simulink model "Closed_loop_BPS_PID_Controller"  (R2023b)
settings: Solver=VariableStepAuto  StartTime=0.0  StopTime=10  RelTol=1e-3
libraries: simulink x2, simulink_extras x2, mcbcontrolslib x2, dspstat3 x2, slpidlib x2
settings Model: Creator=msdbg  LastModifiedBy=msdbg

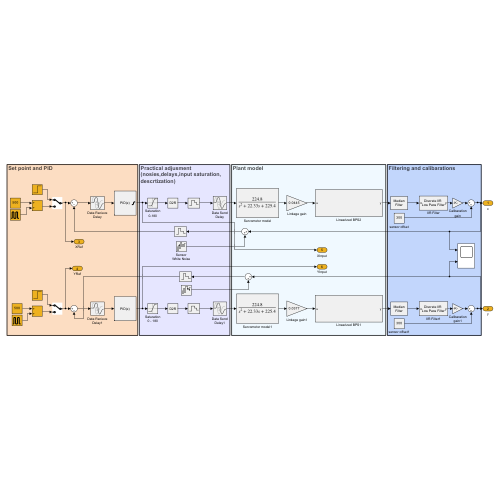
[thumbnail: Simulink's stored preview of the top-level diagram]
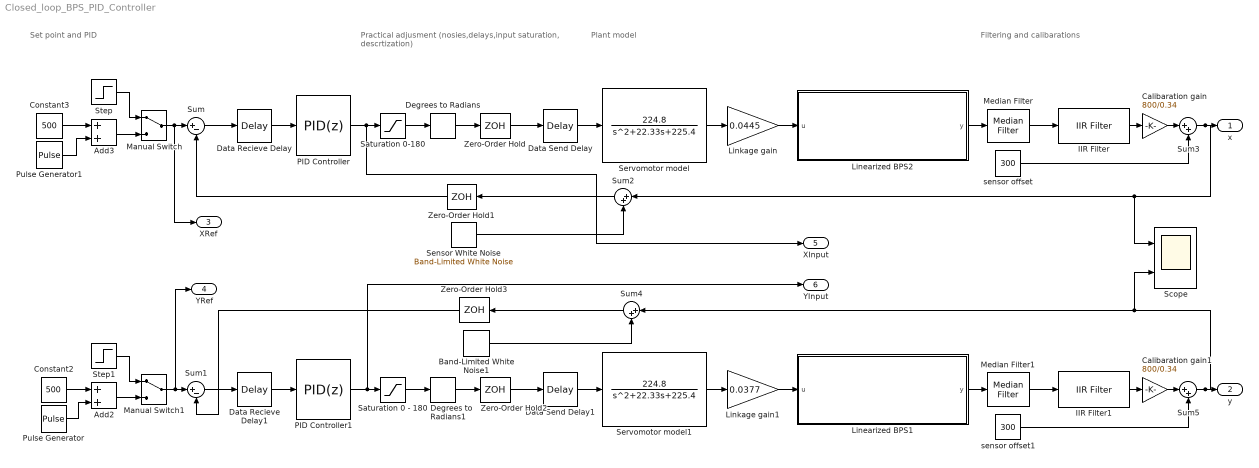
== system Closed_loop_BPS_PID_Controller ==
  note: Set point and PID
  note: Filtering and calibarations
  note: Plant model
  note: Practical adjusment
      | (nosies,delays,input saturation,
      | descrtization)
  Add2 : Sum
  Add3 : Sum
  Band-Limited White Noise1 : simulink/Sources/Band-Limited White Noise  Cov=[0.1]  Ts=0.1  seed=[23341]
  Calibaration gain : Gain  Gain=800/0.34
  Calibaration gain1 : Gain  Gain=800/0.34
  Constant2 : Constant  Value=500
  Constant3 : Constant  Value=500
  Data Recieve Delay : TransportDelay  DelayTime=0.05
  Data Recieve Delay1 : TransportDelay  DelayTime=0.05
  Data Send Delay : TransportDelay  DelayTime=0.05
  Data Send Delay1 : TransportDelay  DelayTime=0.05
  Degrees to Radians : simulink_extras/Transformations/Degrees to Radians
  Degrees to Radians1 : simulink_extras/Transformations/Degrees to Radians
  IIR Filter : mcbcontrolslib/IIR Filter  VariantControl=Low Pass Filter  VariantSelect=Low-pass  Filter_constant=0.7  advancedSettings=off  Ts=50e-6  cutOff_freq=7427.2307
      settings: LibrarySourceBlock=mcblib/Signal Management/IIR Filter
  IIR Filter1 : mcbcontrolslib/IIR Filter  VariantControl=Low Pass Filter  VariantSelect=Low-pass  Filter_constant=0.7  advancedSettings=off  Ts=50e-6  cutOff_freq=7427.2307
      settings: LibrarySourceBlock=mcblib/Signal Management/IIR Filter
  Linearized BPS1 : Subsystem
  Linearized BPS2 : Subsystem
  Linkage gain : Gain  Gain=0.0445
  Linkage gain1 : Gain  Gain=0.0377
  Manual Switch : ManualSwitch
  Manual Switch1 : ManualSwitch
  Median Filter : dspstat3/Median Filter  WindowLength=3  SimulateUsing=Interpreted execution
      settings: LibrarySourceBlock=|
      | dspfdesign/Median
      | Filter
  Median Filter1 : dspstat3/Median Filter  WindowLength=3  SimulateUsing=Interpreted execution
      settings: LibrarySourceBlock=|
      | dspfdesign/Median
      | Filter
  PID Controller : slpidlib/PID Controller  Controller=PID  Form=Parallel  TimeDomain=Discrete-time  UseExternalTs=off  SampleTime=0.1  IntegratorMethod=Forward Euler  FilterMethod=Forward Euler  ControllerParametersSource=internal  P=0.105  I=0.00084  UseKiTs=off  D=0.09  N=12  UseFilter=off  TunerSelectOption=Transfer Function Based (PID Tuner App)  InitialConditionSource=internal  InitialConditionForIntegrator=0  InitialConditionForFilter=0  DifferentiatorICPrevScaledInput=0  ExternalReset=none  TrackingMode=off  Kt=1  LimitOutput=on  SatLimitsSource=internal  UpperSaturationLimit=90  LowerSaturationLimit=-90  LinearizeAsGain=on  AntiWindupMode=clamping  Kb=1  LimitIntegrator=off  UpperIntegratorSaturationLimit=inf  LowerIntegratorSaturationLimit=-inf  POutMin=[]  POutMax=[]  IOutMin=[]  IOutMax=[]  DOutMin=[]  DOutMax=[]  NOutMin=[]  NOutMax=[]  SumOutMin=[]  SumOutMax=[]  SaturationOutMin=[]  SaturationOutMax=[]  PParamMin=[]  PParamMax=[]  IParamMin=[]  IParamMax=[]  DParamMin=[]  DParamMax=[]  NParamMin=[]  NParamMax=[]  KbParamMin=[]  KbParamMax=[]  KtParamMin=[]  KtParamMax=[]  KbOutMin=[]  KbOutMax=[]  KtOutMin=[]  KtOutMax=[]  IntegratorOutMin=[]  IntegratorOutMax=[]  FilterOutMin=[]  FilterOutMax=[]  SumI1OutMin=[]  SumI1OutMax=[]  SumI2OutMin=[]  SumI2OutMax=[]  SumI3OutMin=[]  SumI3OutMax=[]  SumI4OutMin=[]  SumI4OutMax=[]  SumDOutMin=[]  SumDOutMax=[]  DifferentiatorOutMin=[]  DifferentiatorOutMax=[]  FilterDiffOutCoefMin=[]  FilterDiffOutCoefMax=[]  ReciprocalOutMin=[]  ReciprocalOutMax=[]  SumDenOutMin=[]  SumDenOutMax=[]  SumNumOutMin=[]  SumNumOutMax=[]  DivideOutMin=[]  DivideOutMax=[]  UdiffTsProdOutMin=[]  UdiffTsProdOutMax=[]  NTsProdOutMin=[]  NTsProdOutMax=[]  UintegralTsProdOutMin=[]  UintegralTsProdOutMax=[]  UngainTsProdOutMin=[]  UngainTsProdOutMax=[]  ClampingZeroOutDataTypeStr=Inherit: Inherit via back propagation  ClampingZeroOutMin=[]  ClampingZeroOutMax=[]  FilterDenConstantOutDataTypeStr=Inherit: Inherit via back propagation  FilterDenConstantOutMin=[]  FilterDenConstantOutMax=[]  PCopyOutDataTypeStr=Inherit: Inherit via back propagation  PCopyOutMin=[]  PCopyOutMax=[]  NCopyOutDataTypeStr=Inherit: Inherit via back propagation  NCopyOutMin=[]  NCopyOutMax=[]  IntegratorContinuousStateAttributes=''  IntegratorStateMustResolveToSignalObject=off  IntegratorRTWStateStorageClass=Auto  FilterContinuousStateAttributes=''  FilterStateMustResolveToSignalObject=off  FilterRTWStateStorageClass=Auto  ParallelPVariant=InternalParameters  IdealPVariant=Disabled  IVariant=InternalParameters  DVariant=InternalParameters  IntegratorVariant=Discrete  SatVariant=Enabled  AWVariant=DiscClampingParallel  PCopyVariant=Disabled  TRVariant=Disabled  FdbkBlocksVariant=Forward  IdealPFdbkVariant=Disabled  SatFdbkVariant=Disabled  DerivativeFilterVariant=Differentiator  NVariant=Passthrough  NCopyVariant=Disabled_SignalSpec  FilterICVariant=InternalICsDifferentiator  IntegratorICVariant=InternalICs  ExternalResetVariant=Disabled  TRSumVariant=Passthrough  SumFdbkVariant=Disabled  SumVariant=Sum_PID  TsampFilterVariant=InternalTs  TsampNgainVariant=Passthrough  TsampIntegralVariant=Disabled_SignalSpec  ExternalSaturationOutDataTypeStr=Inherit: Same as second input
  PID Controller1 : slpidlib/PID Controller  Controller=PID  Form=Parallel  TimeDomain=Discrete-time  UseExternalTs=off  SampleTime=0.1  IntegratorMethod=Forward Euler  FilterMethod=Forward Euler  ControllerParametersSource=internal  P=0.107  I=0.00184  UseKiTs=off  D=0.089  N=5  UseFilter=off  TunerSelectOption=Transfer Function Based (PID Tuner App)  InitialConditionSource=internal  InitialConditionForIntegrator=0  InitialConditionForFilter=0  DifferentiatorICPrevScaledInput=0  ExternalReset=none  TrackingMode=off  Kt=1  LimitOutput=off  SatLimitsSource=internal  UpperSaturationLimit=180  LowerSaturationLimit=0  LinearizeAsGain=on  AntiWindupMode=clamping  Kb=1  LimitIntegrator=off  UpperIntegratorSaturationLimit=inf  LowerIntegratorSaturationLimit=-inf  POutMin=[]  POutMax=[]  IOutMin=[]  IOutMax=[]  DOutMin=[]  DOutMax=[]  NOutMin=[]  NOutMax=[]  SumOutMin=[]  SumOutMax=[]  SaturationOutMin=[]  SaturationOutMax=[]  PParamMin=[]  PParamMax=[]  IParamMin=[]  IParamMax=[]  DParamMin=[]  DParamMax=[]  NParamMin=[]  NParamMax=[]  KbParamMin=[]  KbParamMax=[]  KtParamMin=[]  KtParamMax=[]  KbOutMin=[]  KbOutMax=[]  KtOutMin=[]  KtOutMax=[]  IntegratorOutMin=[]  IntegratorOutMax=[]  FilterOutMin=[]  FilterOutMax=[]  SumI1OutMin=[]  SumI1OutMax=[]  SumI2OutMin=[]  SumI2OutMax=[]  SumI3OutMin=[]  SumI3OutMax=[]  SumI4OutMin=[]  SumI4OutMax=[]  SumDOutMin=[]  SumDOutMax=[]  DifferentiatorOutMin=[]  DifferentiatorOutMax=[]  FilterDiffOutCoefMin=[]  FilterDiffOutCoefMax=[]  ReciprocalOutMin=[]  ReciprocalOutMax=[]  SumDenOutMin=[]  SumDenOutMax=[]  SumNumOutMin=[]  SumNumOutMax=[]  DivideOutMin=[]  DivideOutMax=[]  UdiffTsProdOutMin=[]  UdiffTsProdOutMax=[]  NTsProdOutMin=[]  NTsProdOutMax=[]  UintegralTsProdOutMin=[]  UintegralTsProdOutMax=[]  UngainTsProdOutMin=[]  UngainTsProdOutMax=[]  ClampingZeroOutDataTypeStr=Inherit: Inherit via back propagation  ClampingZeroOutMin=[]  ClampingZeroOutMax=[]  FilterDenConstantOutDataTypeStr=Inherit: Inherit via back propagation  FilterDenConstantOutMin=[]  FilterDenConstantOutMax=[]  PCopyOutDataTypeStr=Inherit: Inherit via back propagation  PCopyOutMin=[]  PCopyOutMax=[]  NCopyOutDataTypeStr=Inherit: Inherit via back propagation  NCopyOutMin=[]  NCopyOutMax=[]  IntegratorContinuousStateAttributes=''  IntegratorStateMustResolveToSignalObject=off  IntegratorRTWStateStorageClass=Auto  FilterContinuousStateAttributes=''  FilterStateMustResolveToSignalObject=off  FilterRTWStateStorageClass=Auto  ParallelPVariant=InternalParameters  IdealPVariant=Disabled  IVariant=InternalParameters  DVariant=InternalParameters  IntegratorVariant=Discrete  SatVariant=Disabled  AWVariant=Passthrough  PCopyVariant=Disabled  TRVariant=Disabled  FdbkBlocksVariant=Forward  IdealPFdbkVariant=Disabled  SatFdbkVariant=Disabled  DerivativeFilterVariant=Differentiator  NVariant=Passthrough  NCopyVariant=Disabled_SignalSpec  FilterICVariant=InternalICsDifferentiator  IntegratorICVariant=InternalICs  ExternalResetVariant=Disabled  TRSumVariant=Passthrough  SumFdbkVariant=Disabled  SumVariant=Sum_PID  TsampFilterVariant=InternalTs  TsampNgainVariant=Passthrough  TsampIntegralVariant=Disabled_SignalSpec  ExternalSaturationOutDataTypeStr=Inherit: Same as second input
  Pulse Generator : DiscretePulseGenerator  PulseType=Time based  Amplitude=100  Period=20  PulseWidth=50  PhaseDelay=2.5
  Pulse Generator1 : DiscretePulseGenerator  PulseType=Time based  Amplitude=100  Period=20  PulseWidth=50
  Saturation 0 - 180 : Saturate  UpperLimit=90  LowerLimit=-90
  Saturation 0-180 : Saturate  UpperLimit=90  LowerLimit=-90
  Scope : Scope  NumInputPorts=2
  Sensor White Noise : simulink/Sources/Band-Limited White Noise  Cov=[0.7]  Ts=0.1  seed=[23341]
  Servomotor model : TransferFcn  Numerator=[224.8]  Denominator=[1 22.33 225.4]
  Servomotor model1 : TransferFcn  Numerator=[224.8]  Denominator=[1 22.33 225.4]
  Step : Step  Time=0  After=550  SampleTime=0
  Step1 : Step  Time=0  After=550  SampleTime=0
  Sum : Sum  Inputs=|+-
  Sum1 : Sum  Inputs=|+-
  Sum{2..5} (4 alike) : Sum  Inputs=|++
  Zero-Order Hold : ZeroOrderHold  SampleTime=0.1
  Zero-Order Hold1 : ZeroOrderHold  SampleTime=0.033
  Zero-Order Hold2 : ZeroOrderHold  SampleTime=0.08
  Zero-Order Hold3 : ZeroOrderHold  SampleTime=0.05
  sensor offset : Constant  Value=300
  sensor offset1 : Constant  Value=300
  x : Outport
  y : Outport  Port=2
  XRef : Outport  Port=3
  YRef : Outport  Port=4
  XInput : Outport  Port=5
  YInput : Outport  Port=6
  wires:
  Servomotor model/1 -> Linkage gain/1
  Linkage gain/1 -> Linearized BPS2/1(u)
  Sum/1 -> Data Recieve Delay/1
  Manual Switch/1 -> XRef/1, Sum/1
  Step/1 -> Manual Switch/1
  Saturation 0-180/1 -> Degrees to Radians/1
  Zero-Order Hold/1 -> Data Send Delay/1
  Sum2/1 -> Zero-Order Hold1/1
  Zero-Order Hold1/1 -> Sum/2
  Data Recieve Delay/1 -> PID Controller/1
  Sensor White Noise/1 -> Sum2/2
  Linearized BPS2/1(y) -> Median Filter/1
  Sum3/1 -> Scope/1, Sum2/1, x/1
  sensor offset/1 -> Sum3/2
  Data Send Delay/1 -> Servomotor model/1
  IIR Filter/1 -> Calibaration gain/1
  Calibaration gain/1 -> Sum3/1
  Degrees to Radians/1 -> Zero-Order Hold/1
  Median Filter/1 -> IIR Filter/1
  Sum5/1 -> Scope/2, Sum4/1, y/1
  IIR Filter1/1 -> Calibaration gain1/1
  Median Filter1/1 -> IIR Filter1/1
  Calibaration gain1/1 -> Sum5/1
  Saturation 0 - 180/1 -> Degrees to Radians1/1
  Linearized BPS1/1(y) -> Median Filter1/1
  sensor offset1/1 -> Sum5/2
  Band-Limited White Noise1/1 -> Sum4/2
  Data Send Delay1/1 -> Servomotor model1/1
  Zero-Order Hold2/1 -> Data Send Delay1/1
  Zero-Order Hold3/1 -> Sum1/2
  Sum1/1 -> Data Recieve Delay1/1
  Data Recieve Delay1/1 -> PID Controller1/1
  Sum4/1 -> Zero-Order Hold3/1
  Degrees to Radians1/1 -> Zero-Order Hold2/1
  Step1/1 -> Manual Switch1/1
  Linkage gain1/1 -> Linearized BPS1/1(u)
  Manual Switch1/1 -> YRef/1, Sum1/1
  Servomotor model1/1 -> Linkage gain1/1
  Add2/1 -> Manual Switch1/2
  Add3/1 -> Manual Switch/2
  Constant3/1 -> Add3/1
  Pulse Generator/1 -> Add2/2
  Constant2/1 -> Add2/1
  Pulse Generator1/1 -> Add3/2
  PID Controller1/1 -> YInput/1, Saturation 0 - 180/1
  PID Controller/1 -> XInput/1, Saturation 0-180/1

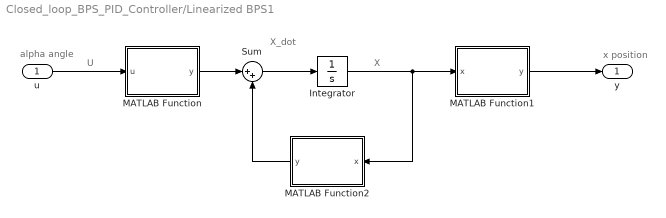
== system Closed_loop_BPS_PID_Controller/Linearized BPS1 ==
  note: x position
  note: alpha angle
  note: X
  note: X_dot
  note: U
  u : Inport
  Integrator : Integrator
  MATLAB Function : MATLAB Function  TreatAsAtomicUnit=on
  MATLAB Function1 : MATLAB Function  TreatAsAtomicUnit=on
  MATLAB Function2 : MATLAB Function  TreatAsAtomicUnit=on
  Sum : Sum  Inputs=|++
  y : Outport
  wires:
  Sum/1 -> Integrator/1
  Integrator/1 -> MATLAB Function2/1(x), MATLAB Function1/1(x)
  MATLAB Function/1(y) -> Sum/1
  u/1 -> MATLAB Function/1(u)
  MATLAB Function2/1(y) -> Sum/2
  MATLAB Function1/1(y) -> y/1

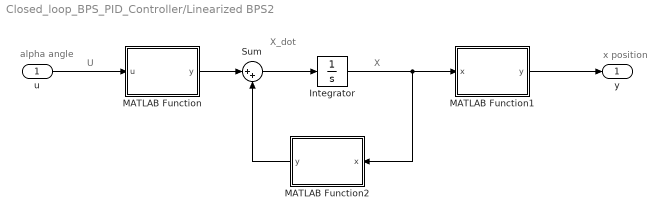
== system Closed_loop_BPS_PID_Controller/Linearized BPS2 ==
  note: x position
  note: alpha angle
  note: X
  note: X_dot
  note: U
  u : Inport
  Integrator : Integrator
  MATLAB Function : MATLAB Function  TreatAsAtomicUnit=on
  MATLAB Function1 : MATLAB Function  TreatAsAtomicUnit=on
  MATLAB Function2 : MATLAB Function  TreatAsAtomicUnit=on
  Sum : Sum  Inputs=|++
  y : Outport
  wires:
  Sum/1 -> Integrator/1
  Integrator/1 -> MATLAB Function2/1(x), MATLAB Function1/1(x)
  MATLAB Function/1(y) -> Sum/1
  u/1 -> MATLAB Function/1(u)
  MATLAB Function2/1(y) -> Sum/2
  MATLAB Function1/1(y) -> y/1

== matlab function Closed_loop_BPS_PID_Controller/Linearized BPS2/MATLAB Function1 ==
  data: x input size=[2 1]; y output
function y = C(x)

y = [1 0]*x;

== matlab function Closed_loop_BPS_PID_Controller/Linearized BPS2/MATLAB Function2 ==
  data: x input size=[2 1]; y output size=[2 1]
function y = A(x)

y = [0 1 ; 0 0]*x;

== matlab function Closed_loop_BPS_PID_Controller/Linearized BPS1/MATLAB Function ==
  data: u input; y output
function y = B(u)

y = [0; 5/7*9.81]*u;

== matlab function Closed_loop_BPS_PID_Controller/Linearized BPS1/MATLAB Function1 ==
  data: x input size=[2 1]; y output
function y = C(x)

y = [1 0]*x;

== matlab function Closed_loop_BPS_PID_Controller/Linearized BPS1/MATLAB Function2 ==
  data: x input size=[2 1]; y output size=[2 1]
function y = A(x)

y = [0 1 ; 0 0]*x;

== matlab function Closed_loop_BPS_PID_Controller/Linearized BPS2/MATLAB Function ==
  data: u input; y output
function y = B(u)

y = [0; 5/7*9.81]*u;
